simulink model "drone_6dof"  (R2020b)
settings: Solver=VariableStepAuto  StartTime=0.0  StopTime=10  RelTol=1e-3
undefined symbols (not defined in the file or in its folder): controller, dynamics, phi0, psi0, theta0, x0, y0, z0
libraries: shared6dof x1
settings Model: Creator=rudog  LastModifiedBy=acnau

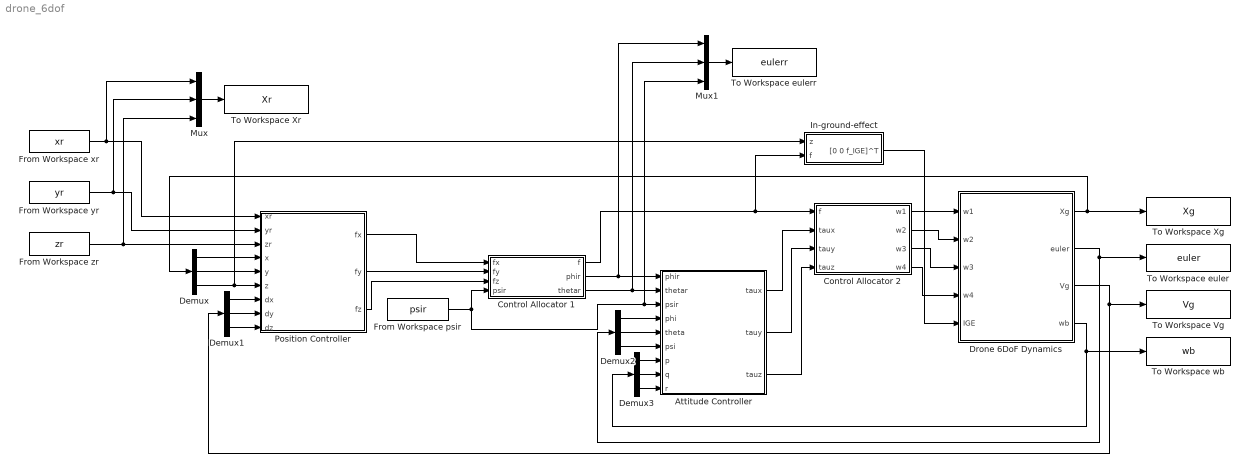
== system drone_6dof ==
  Attitude Controller : Subsystem
  Control Allocator 1 : Subsystem
  Control Allocator 2 : Subsystem
  Demux{,1..3} (4 alike) : Demux  Outputs=3
  Drone 6DoF Dynamics : Subsystem
  From Workspace psir : FromWorkspace  VariableName=psir
  From Workspace xr : FromWorkspace  VariableName=xr
  From Workspace yr : FromWorkspace  VariableName=yr
  From Workspace zr : FromWorkspace  VariableName=zr
  In-ground-effect : Subsystem
  Mux : Mux  Inputs=3
  Mux1 : Mux  Inputs=3
  Position Controller : Subsystem
  To Workspace Vg : ToWorkspace  VariableName=Vg  SaveFormat=Structure With Time  SampleTime=-1
  To Workspace Xg : ToWorkspace  VariableName=Xg  SaveFormat=Structure With Time  SampleTime=-1
  To Workspace Xr : ToWorkspace  VariableName=Xr  SaveFormat=Structure With Time  SampleTime=-1
  To Workspace euler : ToWorkspace  VariableName=euler  SaveFormat=Structure With Time  SampleTime=-1
  To Workspace eulerr : ToWorkspace  VariableName=eulerr  SaveFormat=Structure With Time  SampleTime=-1
  To Workspace wb : ToWorkspace  VariableName=wb  SaveFormat=Structure With Time  SampleTime=-1
  wires:
  Position Controller/1(fx) -> Control Allocator 1/1(fx)
  Position Controller/2(fy) -> Control Allocator 1/2(fy)
  Position Controller/3(fz) -> Control Allocator 1/3(fz)
  Demux/1 -> Position Controller/4(x)
  Demux/2 -> Position Controller/5(y)
  Demux1/1 -> Position Controller/7(dx)
  Demux1/2 -> Position Controller/8(dy)
  Demux1/3 -> Position Controller/9(dz)
  Demux2/1 -> Attitude Controller/4(phi)
  Demux2/2 -> Attitude Controller/5(theta)
  Demux2/3 -> Attitude Controller/6(psi)
  Demux3/1 -> Attitude Controller/7(p)
  Demux3/2 -> Attitude Controller/8(q)
  Demux3/3 -> Attitude Controller/9(r)
  From Workspace zr/1 -> Mux/3, Position Controller/3(zr)
  From Workspace yr/1 -> Mux/2, Position Controller/2(yr)
  From Workspace xr/1 -> Mux/1, Position Controller/1(xr)
  Control Allocator 2/1(w1) -> Drone 6DoF Dynamics/1(w1)
  Control Allocator 2/2(w2) -> Drone 6DoF Dynamics/2(w2)
  Control Allocator 2/3(w3) -> Drone 6DoF Dynamics/3(w3)
  Control Allocator 2/4(w4) -> Drone 6DoF Dynamics/4(w4)
  Attitude Controller/1(taux) -> Control Allocator 2/2(taux)
  Attitude Controller/2(tauy) -> Control Allocator 2/3(tauy)
  Attitude Controller/3(tauz) -> Control Allocator 2/4(tauz)
  Drone 6DoF Dynamics/2(euler) -> Demux2/1, To Workspace euler/1
  Drone 6DoF Dynamics/3(Vg) -> Demux1/1, To Workspace Vg/1
  Drone 6DoF Dynamics/4(wb) -> Demux3/1, To Workspace wb/1
  Drone 6DoF Dynamics/1(Xg) -> To Workspace Xg/1, Demux/1
  Mux/1 -> To Workspace Xr/1
  Control Allocator 1/2(phir) -> Mux1/1, Attitude Controller/1(phir)
  Control Allocator 1/3(thetar) -> Mux1/2, Attitude Controller/2(thetar)
  From Workspace psir/1 -> Mux1/3, Attitude Controller/3(psir), Control Allocator 1/4(psir)
  Mux1/1 -> To Workspace eulerr/1
  Demux/3 -> In-ground-effect/1(z), Position Controller/6(z)
  Control Allocator 1/1(f) -> In-ground-effect/2(f), Control Allocator 2/1(f)
  In-ground-effect/1("[0 0 f_IGE]^T") -> Drone 6DoF Dynamics/5(IGE)

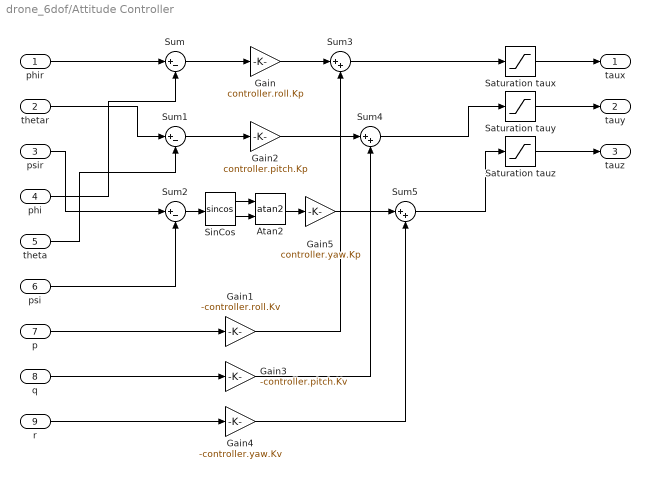
== system drone_6dof/Attitude Controller ==
  phir : Inport
  thetar : Inport  Port=2
  psir : Inport  Port=3
  phi : Inport  Port=4
  theta : Inport  Port=5
  psi : Inport  Port=6
  p : Inport  Port=7
  q : Inport  Port=8
  r : Inport  Port=9
  Atan2 : Trigonometry  Operator=atan2
  Gain : Gain  Gain=controller.roll.Kp
  Gain1 : Gain  Gain=-controller.roll.Kv
  Gain2 : Gain  Gain=controller.pitch.Kp
  Gain3 : Gain  Gain=-controller.pitch.Kv
  Gain4 : Gain  Gain=-controller.yaw.Kv
  Gain5 : Gain  Gain=controller.yaw.Kp
  Saturation taux : Saturate  UpperLimit=controller.roll.tauMax  LowerLimit=controller.roll.tauMin
  Saturation tauy : Saturate  UpperLimit=controller.pitch.tauMax  LowerLimit=controller.pitch.tauMin
  Saturation tauz : Saturate  UpperLimit=controller.yaw.tauMax  LowerLimit=controller.yaw.tauMin
  SinCos : Trigonometry  Operator=sincos
  Sum : Sum  Inputs=|+-
  Sum1 : Sum  Inputs=|+-
  Sum2 : Sum  Inputs=|+-
  Sum3 : Sum  Inputs=|++
  Sum4 : Sum  Inputs=|++
  Sum5 : Sum  Inputs=|++
  taux : Outport
  tauy : Outport  Port=2
  tauz : Outport  Port=3
  wires:
  phir/1 -> Sum/1
  phi/1 -> Sum/2
  thetar/1 -> Sum1/1
  theta/1 -> Sum1/2
  psir/1 -> Sum2/1
  psi/1 -> Sum2/2
  p/1 -> Gain1/1
  Sum/1 -> Gain/1
  Gain/1 -> Sum3/1
  Gain1/1 -> Sum3/2
  q/1 -> Gain3/1
  r/1 -> Gain4/1
  Sum1/1 -> Gain2/1
  Gain2/1 -> Sum4/1
  Gain3/1 -> Sum4/2
  Gain4/1 -> Sum5/2
  Gain5/1 -> Sum5/1
  Sum3/1 -> Saturation taux/1
  Sum4/1 -> Saturation tauy/1
  Sum5/1 -> Saturation tauz/1
  Saturation taux/1 -> taux/1
  Saturation tauy/1 -> tauy/1
  Saturation tauz/1 -> tauz/1
  Sum2/1 -> SinCos/1
  SinCos/1 -> Atan2/1
  SinCos/2 -> Atan2/2
  Atan2/1 -> Gain5/1

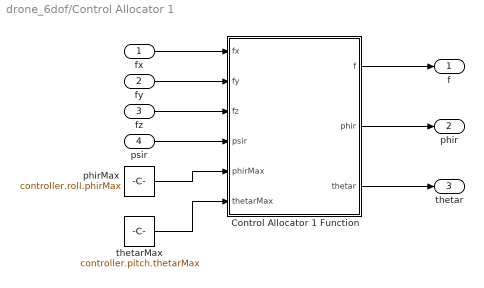
== system drone_6dof/Control Allocator 1 ==
  fx : Inport
  fy : Inport  Port=2
  fz : Inport  Port=3
  psir : Inport  Port=4
  Control Allocator 1 Function : MATLAB Function  TreatAsAtomicUnit=on
  phirMax : Constant  Value=controller.roll.phirMax
  thetarMax : Constant  Value=controller.pitch.thetarMax
  f : Outport
  phir : Outport  Port=2
  thetar : Outport  Port=3
  wires:
  fx/1 -> Control Allocator 1 Function/1(fx)
  fy/1 -> Control Allocator 1 Function/2(fy)
  fz/1 -> Control Allocator 1 Function/3(fz)
  psir/1 -> Control Allocator 1 Function/4(psir)
  Control Allocator 1 Function/1(f) -> f/1
  Control Allocator 1 Function/2(phir) -> phir/1
  Control Allocator 1 Function/3(thetar) -> thetar/1
  phirMax/1 -> Control Allocator 1 Function/5(phirMax)
  thetarMax/1 -> Control Allocator 1 Function/6(thetarMax)

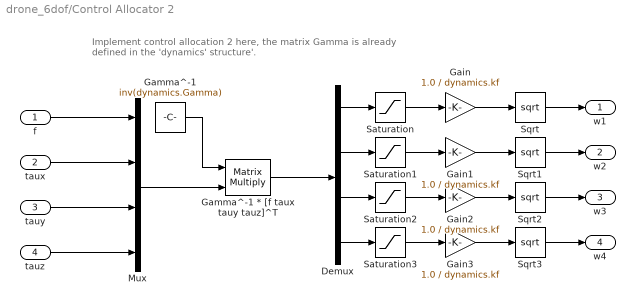
== system drone_6dof/Control Allocator 2 ==
  note: Implement control allocation 2 here, the matrix Gamma is already
      | defined in the 'dynamics' structure'.
  f : Inport
  taux : Inport  Port=2
  tauy : Inport  Port=3
  tauz : Inport  Port=4
  Demux : Demux
  Gain{,1..3} (4 alike) : Gain  Gain=1.0 / dynamics.kf
  Gamma^-1 : Constant  Value=inv(dynamics.Gamma)
  Gamma^-1 * [f taux tauy tauz]^T : Product  Multiplication=Matrix(*)
  Mux : Mux
  Saturation{,1..3} (4 alike) : Saturate  UpperLimit=inf  LowerLimit=0
  Sqrt{,1..3} (4 alike) : Sqrt  SaturateOnIntegerOverflow=on
  w1 : Outport
  w2 : Outport  Port=2
  w3 : Outport  Port=3
  w4 : Outport  Port=4
  wires:
  f/1 -> Mux/1
  taux/1 -> Mux/2
  tauy/1 -> Mux/3
  tauz/1 -> Mux/4
  Mux/1 -> Gamma^-1 * [f taux tauy tauz]^T/2
  Gamma^-1/1 -> Gamma^-1 * [f taux tauy tauz]^T/1
  Gamma^-1 * [f taux tauy tauz]^T/1 -> Demux/1
  Demux/1 -> Saturation/1
  Demux/2 -> Saturation1/1
  Demux/3 -> Saturation2/1
  Demux/4 -> Saturation3/1
  Gain/1 -> Sqrt/1
  Gain1/1 -> Sqrt1/1
  Gain2/1 -> Sqrt2/1
  Gain3/1 -> Sqrt3/1
  Sqrt/1 -> w1/1
  Sqrt1/1 -> w2/1
  Sqrt2/1 -> w3/1
  Sqrt3/1 -> w4/1
  Saturation/1 -> Gain/1
  Saturation1/1 -> Gain1/1
  Saturation2/1 -> Gain2/1
  Saturation3/1 -> Gain3/1

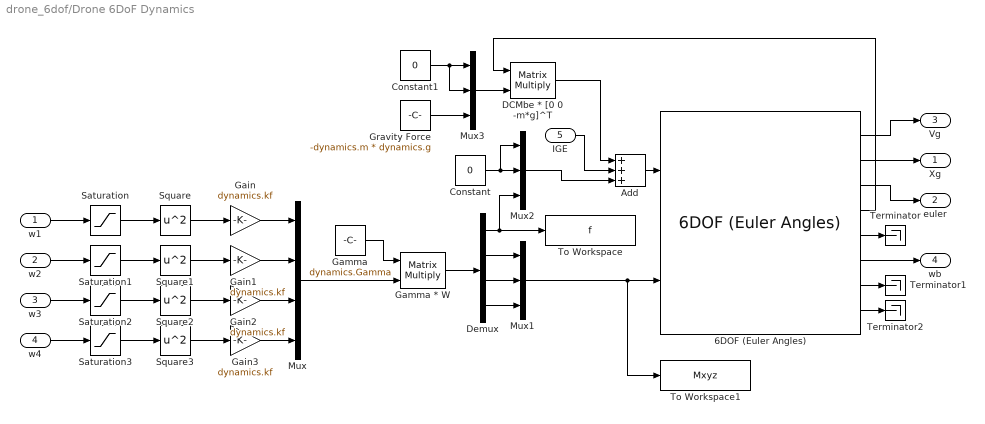
== system drone_6dof/Drone 6DoF Dynamics ==
  w1 : Inport
  w2 : Inport  Port=2
  w3 : Inport  Port=3
  w4 : Inport  Port=4
  IGE : Inport  Port=5
  6DOF (Euler Angles) : shared6dof/6DOF (Euler Angles)  units=Metric (MKS)  mtype=Fixed  rep=Euler Angles  xme_0=[x0, y0, z0]  Vm_0=[0 0 0]  eul_0=[phi0, theta0, psi0]  pm_0=[0 0 0]  mass_0=dynamics.m  mass_e=0.5  mass_f=2.0  inertia=dynamics.J  inertia_e=eye(3)  inertia_f=2*eye(3)  k_quat=1.0  vre_flag=on  abi_flag=off  aMode=0  xme_statename=''  Vm_statename=''  eul_statename=''  quat_statename=''  pm_statename=''  mass_statename=''
      settings: SourceProductBaseCode=AE,PW,MT,UV,VE,VP
  Add : Sum  Inputs=+++
  Constant : Constant  Value=0
  Constant1 : Constant  Value=0
  DCMbe * [0 0 -m*g]^T : Product  Multiplication=Matrix(*)
  Demux : Demux
  Gain{,1..3} (4 alike) : Gain  Gain=dynamics.kf
  Gamma : Constant  Value=dynamics.Gamma
  Gamma * W : Product  Multiplication=Matrix(*)
  Gravity Force : Constant  Value=-dynamics.m * dynamics.g
  Mux : Mux
  Mux1 : Mux  Inputs=3
  Mux2 : Mux  Inputs=3
  Mux3 : Mux  Inputs=3
  Saturation{,1..3} (4 alike) : Saturate  UpperLimit=dynamics.wMax  LowerLimit=dynamics.wMin
  Square{,1..3} (4 alike) : Math  Operator=square  SaturateOnIntegerOverflow=on
  Terminator : Terminator
  Terminator1 : Terminator
  Terminator2 : Terminator
  To Workspace : ToWorkspace  VariableName=f  SaveFormat=Structure With Time  SampleTime=-1
  To Workspace1 : ToWorkspace  VariableName=Mxyz  SaveFormat=Structure With Time  SampleTime=-1
  Xg : Outport
  euler : Outport  Port=2
  Vg : Outport  Port=3
  wb : Outport  Port=4
  wires:
  6DOF (Euler Angles)/2 -> Xg/1
  6DOF (Euler Angles)/1 -> Vg/1
  6DOF (Euler Angles)/3 -> euler/1
  w1/1 -> Saturation/1
  w2/1 -> Saturation1/1
  w3/1 -> Saturation2/1
  w4/1 -> Saturation3/1
  Gamma * W/1 -> Demux/1
  Demux/2 -> Mux1/1
  Demux/3 -> Mux1/2
  Demux/4 -> Mux1/3
  Mux1/1 -> To Workspace1/1, 6DOF (Euler Angles)/2
  Mux/1 -> Gamma * W/2
  Gamma/1 -> Gamma * W/1
  Constant/1 -> Mux2/1, Mux2/2
  Demux/1 -> Mux2/3, To Workspace/1
  Mux2/1 -> Add/3
  6DOF (Euler Angles)/6 -> wb/1
  6DOF (Euler Angles)/5 -> Terminator/1
  6DOF (Euler Angles)/7 -> Terminator1/1
  6DOF (Euler Angles)/8 -> Terminator2/1
  Gravity Force/1 -> Mux3/3
  Mux3/1 -> DCMbe * [0 0 -m*g]^T/2
  6DOF (Euler Angles)/4 -> DCMbe * [0 0 -m*g]^T/1
  Constant1/1 -> Mux3/2, Mux3/1
  Saturation/1 -> Square/1
  Square/1 -> Gain/1
  Gain/1 -> Mux/1
  Gain1/1 -> Mux/2
  Saturation1/1 -> Square1/1
  Saturation2/1 -> Square2/1
  Saturation3/1 -> Square3/1
  Square1/1 -> Gain1/1
  Square2/1 -> Gain2/1
  Square3/1 -> Gain3/1
  Gain2/1 -> Mux/3
  Gain3/1 -> Mux/4
  Add/1 -> 6DOF (Euler Angles)/1
  IGE/1 -> Add/2
  DCMbe * [0 0 -m*g]^T/1 -> Add/1

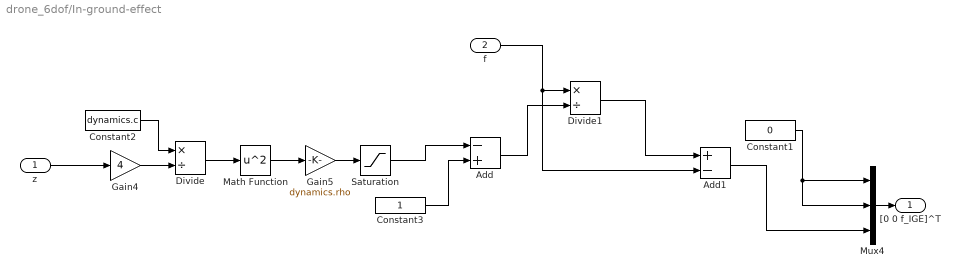
== system drone_6dof/In-ground-effect ==
  z : Inport
  f : Inport  Port=2
  Add : Sum  Inputs=-+
  Add1 : Sum  Inputs=+-
  Constant1 : Constant  Value=0
  Constant2 : Constant  Value=dynamics.c
  Constant3 : Constant
  Divide : Product  Inputs=*/
  Divide1 : Product  Inputs=*/
  Gain4 : Gain  Gain=4
  Gain5 : Gain  Gain=dynamics.rho
  Math Function : Math  Operator=square  SaturateOnIntegerOverflow=on
  Mux4 : Mux  Inputs=3
  Saturation : Saturate  UpperLimit=1  LowerLimit=0
  "[0 0 f_IGE]^T" : Outport
  wires:
  Constant2/1 -> Divide/1
  z/1 -> Gain4/1
  Divide/1 -> Math Function/1
  Gain4/1 -> Divide/2
  Math Function/1 -> Gain5/1
  f/1 -> Add1/2, Divide1/1
  Constant1/1 -> Mux4/1, Mux4/2
  Add/1 -> Divide1/2
  Mux4/1 -> "[0 0 f_IGE]^T"/1
  Saturation/1 -> Add/1
  Constant3/1 -> Add/2
  Gain5/1 -> Saturation/1
  Add1/1 -> Mux4/3
  Divide1/1 -> Add1/1

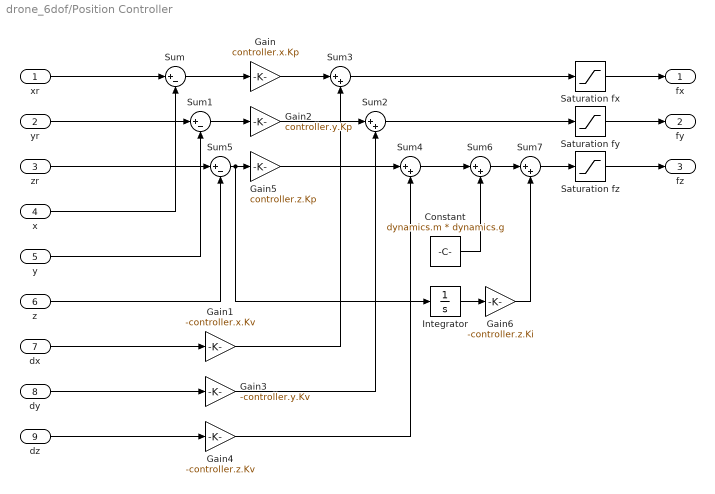
== system drone_6dof/Position Controller ==
  xr : Inport
  yr : Inport  Port=2
  zr : Inport  Port=3
  x : Inport  Port=4
  y : Inport  Port=5
  z : Inport  Port=6
  dx : Inport  Port=7
  dy : Inport  Port=8
  dz : Inport  Port=9
  Constant : Constant  Value=dynamics.m * dynamics.g
  Gain : Gain  Gain=controller.x.Kp
  Gain1 : Gain  Gain=-controller.x.Kv
  Gain2 : Gain  Gain=controller.y.Kp
  Gain3 : Gain  Gain=-controller.y.Kv
  Gain4 : Gain  Gain=-controller.z.Kv
  Gain5 : Gain  Gain=controller.z.Kp
  Gain6 : Gain  Gain=-controller.z.Ki
  Integrator : Integrator
  Saturation fx : Saturate  UpperLimit=controller.x.fMax  LowerLimit=controller.x.fMin
  Saturation fy : Saturate  UpperLimit=controller.y.fMax  LowerLimit=controller.y.fMin
  Saturation fz : Saturate  UpperLimit=controller.z.fMax  LowerLimit=controller.z.fMin
  Sum : Sum  Inputs=|+-
  Sum1 : Sum  Inputs=|+-
  Sum{2..4,6..7} (5 alike) : Sum  Inputs=|++
  Sum5 : Sum  Inputs=|+-
  fx : Outport
  fy : Outport  Port=2
  fz : Outport  Port=3
  wires:
  xr/1 -> Sum/1
  x/1 -> Sum/2
  Sum/1 -> Gain/1
  Gain/1 -> Sum3/1
  dx/1 -> Gain1/1
  Gain1/1 -> Sum3/2
  yr/1 -> Sum1/1
  y/1 -> Sum1/2
  Gain2/1 -> Sum2/1
  dy/1 -> Gain3/1
  dz/1 -> Gain4/1
  Gain3/1 -> Sum2/2
  Sum5/1 -> Integrator/1, Gain5/1
  zr/1 -> Sum5/1
  z/1 -> Sum5/2
  Gain5/1 -> Sum4/1
  Gain4/1 -> Sum4/2
  Sum4/1 -> Sum6/1
  Constant/1 -> Sum6/2
  Saturation fx/1 -> fx/1
  Saturation fy/1 -> fy/1
  Sum6/1 -> Sum7/1
  Sum7/1 -> Saturation fz/1
  Saturation fz/1 -> fz/1
  Sum1/1 -> Gain2/1
  Sum3/1 -> Saturation fx/1
  Integrator/1 -> Gain6/1
  Gain6/1 -> Sum7/2
  Sum2/1 -> Saturation fy/1

== matlab function drone_6dof/Control Allocator 1/Control Allocator 1 Function ==
  data: f output; phir output; thetar output; fx input; fy input; fz input; psir input; phirMax input; thetarMax input
function [f, phir, thetar] = controlAllocator1(fx, fy, fz, psir, phirMax, thetarMax)
% Implement the control allocation 1 here.
% Make sure that all outputs are calculated, see slides for expressions.
% use the commands 'asin' and 'atan2' for arcsine and arctangent computations.
% Check the command 'norm' to compute f
% Dont forget the saturations! Phi and Theta must be inferiorly and
% superiorly saturated. Use phirMax and -phirMax as limits, for example.


f = norm([fx; fy; fz]);

nx = fx / f;
ny = fy / f;
nz = fz / f;

sp = sin(psir);
cp = cos(psir);

phir = asin(nx * sp - ny * cp);
thetar = atan2((nx * cp + ny * sp), nz);

phir = max(-phirMax, min(phirMax, phir));
thetar = max(-thetarMax, min(thetarMax, thetar));


end
